simulink model "PID"  (R2022b)
settings: Solver=FixedStepAuto  StartTime=0.0  StopTime=t_max  FixedStep=timestep  RelTol=1e-3
values from neighbouring files (symbols this model uses):
  denD = sym2poly(denD)    [script.m]
  denU = sym2poly(denU)    [script.m]
  numD = sym2poly(numD)    [script.m]
  numU = sym2poly(numU)    [script.m]
  step_v = 0.4    [script.m]
  timestep = t_max/1e6    (= 0.0015)    [script.m]
undefined symbols (not defined in the file or in its folder): Cd, g, Kp, L, Td, Ti
settings Model: Creator=mluser  LastModifiedBy=mluser

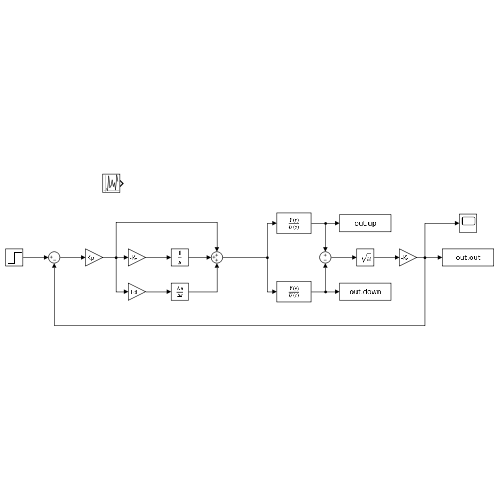
[thumbnail: Simulink's stored preview of the top-level diagram]
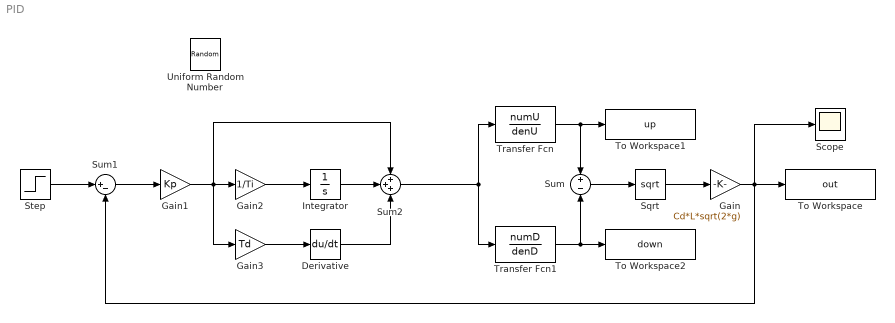
== system PID ==
  Derivative : Derivative
  Gain : Gain  Gain=Cd*L*sqrt(2*g)
  Gain1 : Gain  Gain=Kp
  Gain2 : Gain  Gain=1/Ti
  Gain3 : Gain  Gain=Td
  Integrator : Integrator
  Scope : Scope
  Sqrt : Sqrt
  Step : Step  After=step_v  SampleTime=0
  Sum : Sum  Inputs=+|-
  Sum1 : Sum  Inputs=|+-
  Sum2 : Sum  Inputs=+++
  To Workspace : ToWorkspace  VariableName=out  SampleTime=-1
  To Workspace1 : ToWorkspace  VariableName=up  SampleTime=-1
  To Workspace2 : ToWorkspace  VariableName=down  SampleTime=-1
  Transfer Fcn : TransferFcn  Numerator=numU  Denominator=denU
  Transfer Fcn1 : TransferFcn  Numerator=numD  Denominator=denD
  Uniform Random Number : UniformRandomNumber  SampleTime=timestep
  wires:
  Transfer Fcn/1 -> To Workspace1/1, Sum/1
  Sum/1 -> Sqrt/1
  Sqrt/1 -> Gain/1
  Transfer Fcn1/1 -> To Workspace2/1, Sum/2
  Gain/1 -> Sum1/2, Scope/1, To Workspace/1
  Step/1 -> Sum1/1
  Sum1/1 -> Gain1/1
  Gain3/1 -> Derivative/1
  Gain1/1 -> Gain3/1, Sum2/1, Gain2/1
  Gain2/1 -> Integrator/1
  Integrator/1 -> Sum2/2
  Derivative/1 -> Sum2/3
  Sum2/1 -> Transfer Fcn1/1, Transfer Fcn/1
